simulink model "RM3"  (R2020a)
settings: Solver=ode45  StartTime=0  StopTime=400  FixedStep=0.01  MaxStep=0.01  RelTol=1e-3  EnableMultiTasking=on
values from neighbouring files (symbols this model uses):
  lowerLimitBound = -0.6    [wecSimInputFile.m]
  lowerLimitDamping = 1e3    (= 1000)    [wecSimInputFile.m]
  lowerLimitStiffness = 1e8    (= 100000000)    [wecSimInputFile.m]
  lowerTransitionRegionWidth = 0.1    [wecSimInputFile.m]
  simu = simulationClass()    [wecSimInputFile.m]
  upperLimitBound = 0.6    [wecSimInputFile.m]
  upperLimitDamping = 1e3    (= 1000)    [wecSimInputFile.m]
  upperLimitStiffness = 1e8    (= 100000000)    [wecSimInputFile.m]
  upperTransitionRegionWidth = 0.1    [wecSimInputFile.m]
undefined symbols (not defined in the file or in its folder): body, constraint, pto
libraries: WECSim_Lib x5
settings Model: Creator=mlawson  LastModifiedBy=dforbus
settings SolverCC: ZeroCrossControl=DisableAll  AlgebraicLoopSolver=LineSearch  AutoInsertRateTranBlk=on
settings DataIOCC: SaveFormat=Array  SaveOutput=off  SaveTime=off  ReturnWorkspaceOutputs=off
settings OptimizationCC: LifeSpan=inf  SimCompilerOptimization=on
settings DebuggingCC: UnderspecifiedInitializationDetection=Classic  MergeDetectMultiDrivingBlocksExec=none  SolverPrmCheckMsg=warning  AllowSymbolicDim=off  StateNameClashWarn=warning  SFUnexpectedBacktrackingDiag=warning  SFNoUnconditionalDefaultTransitionDiag=warning  SFExecutionAtInitializationDiag=none  ArithmeticOperatorsInVariantConditions=warning
settings HardwareCC: ProdBitPerPointer=32  ProdBitPerSizeT=32  ProdBitPerPtrDiffT=32  ProdLargestAtomicFloat=None  ProdIntDivRoundTo=Undefined  ProdEndianess=Unspecified  ProdWordSize=32  ProdHWDeviceType=32-bit Generic
settings ModelReferenceCC: PropagateSignalLabelsOutOfModel=off
settings SFSimCC: SimUseLocalCustomCode=off  CustomCodeUndefinedFunction=UseInterfaceOnly
settings RTWCC: RTWUseLocalCustomCode=off
settings CodeAppCC: StateflowObjectComments=on
settings GRTTargetCC: TargetLangStandard=C89/C90 (ANSI)
settings ConfigComp: CovMetricSettings=dw  CovHtmlReporting=on  CovSaveCumulativeToWorkspaceVar=on  CovSaveSingleToWorkspaceVar=on  CovExternalEMLEnable=off  CovSFcnEnable=off
settings SimscapeCC: SimscapeNormalizeSystem=off
settings ConfigurationSet: Description=SimMechanics 2G
settings ExplorerConfigSet: SimMechanicsOpenEditorOnUpdate=off  InternalSimMechanicsExplorerSettings="<ExplorerConfiguration><canonicalview>default</canonicalview><TilePanel><TileInfo><Tiles Columns=\"1\" Count=\"1\" Rows=\"1\"><Column Left=\"2\" Weight=\"1\"/><Column Left=\"1335\"/><Row Top=\"2\" Weight=\"1\"/><Row Top=\"911\"/><Tile Height=\"1\" Width=\"1\" X=\"0\" Y=\"0\"/></Tiles></TileInfo><SceneInfo><SceneViewer><BGColor><R>0.60000002384185791</R><G>0.60000002384185791</G><B>0.60000002384185791</B></BGColor><Camera><Position><X>365.37645888990272</X><Y>-369.82486814446582</Y><Z>359.64809521743916</Z></Position><Center><X>-6.7351450971904585</X><Y>2.2867358426280204</Y><Z>-12.463508769654169</Z></Center><Up><X>-0.40824829046386307</X><Y>0.40824829046386307</Y><Z>0.81649658092772615</Z></Up><Left>-57.820127362122818</Left><Right>57.820127362122818</Right><Bottom>-38.308817187253304</Bottom><Top>38.308817187253304</Top></Camera></SceneViewer></SceneInfo></TilePanel></ExplorerConfiguration>"

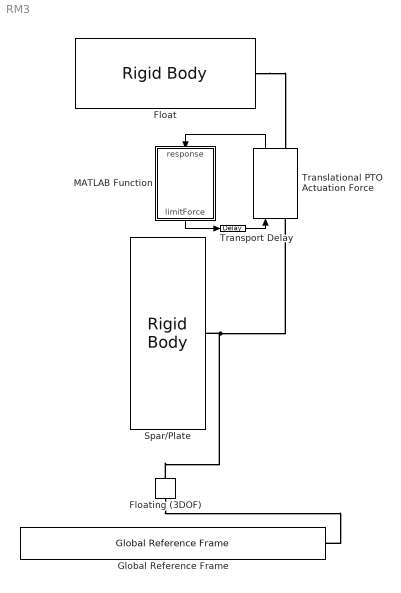
== system RM3 ==
  Float : WECSim_Lib/Body Elements/Rigid Body  body=body(1)
      settings: AttributesFormatString=%<body>  SourceProductName=WEC-Sim
  Floating (3DOF) : WECSim_Lib/Constraints/Floating (3DOF)  constraint=constraint(1)
      settings: AttributesFormatString=%<constraint>  SourceProductName=WEC-Sim
  Global Reference Frame : WECSim_Lib/Frames/Global Reference Frame  waves=waves  simu=simu
      settings: SourceProductName=WEC-Sim
  MATLAB Function : MATLAB Function  TreatAsAtomicUnit=on
  Spar/Plate : WECSim_Lib/Body Elements/Rigid Body  body=body(2)
      settings: AttributesFormatString=%<body>  SourceProductName=WEC-Sim
  Translational PTO Actuation Force : WECSim_Lib/PTOs/Translational PTO Actuation Force  pto=pto(1)
      settings: AttributesFormatString=%<pto>  SourceProductName=WEC-Sim
  Transport Delay : TransportDelay  DelayTime=simu.dt
  wires:
  Translational PTO Actuation Force/1 -> MATLAB Function/1(response)
  MATLAB Function/1(limitForce) -> Transport Delay/1
  Transport Delay/1 -> Translational PTO Actuation Force/1
  connections:
  Floating (3DOF)/LConn1 -- Global Reference Frame/RConn1
  Spar/Plate/RConn1 -- Floating (3DOF)/RConn1 -- Translational PTO Actuation Force/LConn1
  Float/RConn1 -- Translational PTO Actuation Force/RConn1

== matlab function RM3/MATLAB Function ==
  data: response input; limitForce output; upperLimitBound parameter; lowerLimitBound parameter; upperLimitStiffness parameter; lowerLimitStiffness parameter; upperLimitDamping parameter; lowerLimitDamping parameter; upperTransitionRegionWidth parameter; lowerTransitionRegionWidth parameter
function limitForce = limitCalc(response,upperLimitBound, lowerLimitBound,...
upperLimitStiffness, lowerLimitStiffness, upperLimitDamping, lowerLimitDamping,...
upperTransitionRegionWidth, lowerTransitionRegionWidth)

relHeaveDisp = response(3); % relative heave displacement
relHeaveVel = response(9); % relative heave velocity
limitForce = 0; % initialize output force
sForce = 0; % spring force initialize 
dForce = 0; % damping force initialize
frac = 0; % initialize transition region force fraction

if relHeaveDisp > upperLimitBound % check upper limit
    frac = min([1-(((upperLimitBound+upperTransitionRegionWidth) - relHeaveDisp)...
        /(upperTransitionRegionWidth)); 1]); % calculate fraction of limit force, if in transition region
    sForce = -abs(relHeaveDisp - upperLimitBound) * frac * upperLimitStiffness; % spring force in negative direction
    dForce = -relHeaveVel * frac * (relHeaveVel > 0)* upperLimitDamping; % damper force in negative direction iff pos velocity
    limitForce = sForce + dForce; % sum the spring and damper forces
    
elseif relHeaveDisp < lowerLimitBound % check lower limit
    frac = min([1-((relHeaveDisp-(lowerLimitBound-lowerTransitionRegionWidth))/(lowerTransitionRegionWidth)); 1]); % calculate fraction of limit force, if in transition region
    sForce = abs(relHeaveDisp - lowerLimitBound) * frac * lowerLimitStiffness; % spring force in positive direction
    dForce = - relHeaveVel * frac * (relHeaveVel < 0) * lowerLimitDamping; % damper force in positive direction iff neg velocity
    limitForce = sForce + dForce; % sum the spring and damper forces

else 
    limitForce = 0; % no limit force
end

end
